simulink model "Q4_Sensor_Unpack"  (R2018b)
settings: Solver=VariableStepAuto  StartTime=0.0  StopTime=10.0  RelTol=1e-3
(part 1 of 2)
settings Model: Creator=82358  LastModifiedBy=82358

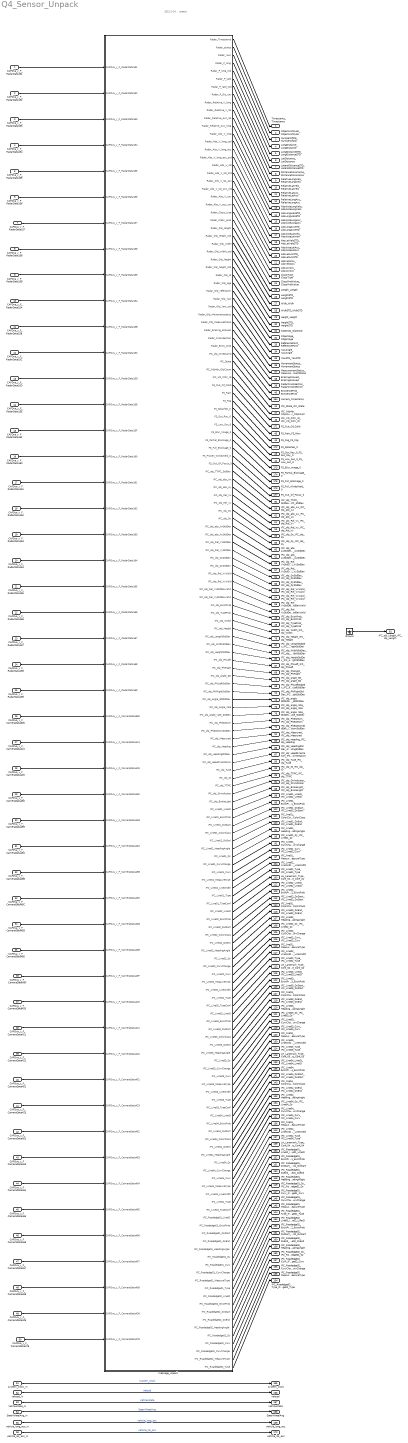
== system Q4_Sensor_Unpack ==
  note: 2021-2-24：unpack
  CAFDva_y_F_RadarData151 : Inport
  CAFDva_y_F_RadarData152 : Inport  Port=2
  CAFDva_y_F_RadarData153 : Inport  Port=3
  CAFDva_y_F_RadarData154 : Inport  Port=4
  CAFDva_y_F_RadarData155 : Inport  Port=5
  CAFDva_y_F_RadarData156 : Inport  Port=6
  CAFDva_y_F_RadarData157 : Inport  Port=7
  CAFDva_y_F_RadarData158 : Inport  Port=8
  CAFDva_y_F_RadarData159 : Inport  Port=9
  CAFDva_y_F_RadarData15A : Inport  Port=10
  CAFDva_y_F_RadarData15B : Inport  Port=11
  CAFDva_y_F_RadarData15C : Inport  Port=12
  CAFDva_y_F_RadarData15D : Inport  Port=13
  CAFDva_y_F_RadarData15E : Inport  Port=14
  CAFDva_y_F_RadarData15F : Inport  Port=15
  CAFDva_y_F_RadarData160 : Inport  Port=16
  CAFDva_y_F_RadarData161 : Inport  Port=17
  CAFDva_y_F_RadarData162 : Inport  Port=18
  CAFDva_y_F_RadarData163 : Inport  Port=19
  CAFDva_y_F_RadarData164 : Inport  Port=20
  CAFDva_y_F_RadarData165 : Inport  Port=21
  CAFDva_y_F_RadarData166 : Inport  Port=22
  CAFDva_y_F_RadarData167 : Inport  Port=23
  CAFDva_y_F_RadarData168 : Inport  Port=24
  CAFDva_y_F_RadarData169 : Inport  Port=25
  CAFDva_y_F_CameraData600 : Inport  Port=26
  CAFDva_y_F_CameraData424 : Inport  Port=27
  CAFDva_y_F_CameraData425 : Inport  Port=28
  CAFDva_y_F_CameraData450 : Inport  Port=29
  CAFDva_y_F_CameraData459 : Inport  Port=30
  CAFDva_y_F_CameraData45A : Inport  Port=31
  CAFDva_y_F_CameraData45B : Inport  Port=32
  CAFDva_y_F_CameraData45C : Inport  Port=33
  CAFDva_y_F_CameraData45D : Inport  Port=34
  CAFDva_y_F_CameraData45E : Inport  Port=35
  CAFDva_y_F_CameraData45F : Inport  Port=36
  CAFDva_y_F_CameraData420 : Inport  Port=37
  CAFDva_y_F_CameraData421 : Inport  Port=38
  CAFDva_y_F_CameraData422 : Inport  Port=39
  CAFDva_y_F_CameraData451 : Inport  Port=40
  CAFDva_y_F_CameraData423 : Inport  Port=41
  CAFDva_y_F_CameraData452 : Inport  Port=42
  CAFDva_y_F_CameraData453 : Inport  Port=43
  CAFDva_y_F_CameraData454 : Inport  Port=44
  CAFDva_y_F_CameraData455 : Inport  Port=45
  CAFDva_y_F_CameraData456 : Inport  Port=46
  CAFDva_y_F_CameraData457 : Inport  Port=47
  CAFDva_y_F_CameraData458 : Inport  Port=48
  CAFDva_y_F_CameraData426 : Inport  Port=49
  CAFDva_y_F_CameraData47E : Inport  Port=50
  system_clock_in : Inport  Port=51  OutDataTypeStr=uint16  PortDimensions=1
  vehspd_in : Inport  Port=52  OutDataTypeStr=T_M_Nm_Float32  PortDimensions=1
  VehYawRate_in : Inport  Port=53  OutDataTypeStr=T_M_Nm_Float32  PortDimensions=1
  SteerWheelAng_in : Inport  Port=54  OutDataTypeStr=T_M_Nm_Float32  PortDimensions=1
  vehicle_long_acc_in : Inport  Port=55  OutDataTypeStr=T_M_Nm_Float32  PortDimensions=1
  vehicle_lat_acc_in : Inport  Port=56  OutDataTypeStr=T_M_Nm_Float32  PortDimensions=1
  Ground : Ground
  message_unpack : MATLAB Function  TreatAsAtomicUnit=on
  Timestamp_Timestamp : Outport
  ObjectListQuali_ObjectListQuali : Outport  Port=2
  NumberOfObj_NumberOfObj : Outport  Port=3
  LongDistance_LongDistance : Outport  Port=4
  LongDistanceSTD_LongDistanceSTD : Outport  Port=5
  LatDistance_LatDistance : Outport  Port=6
  LateralDistanceSTD_LateralDistanceSTD : Outport  Port=7
  DistanceCovariance_DistanceCovariance : Outport  Port=8
  RelativeLongVelo_RelativeLongVelo : Outport  Port=9
  RelativeLatVelo_RelativeLatVelo : Outport  Port=10
  RelativeLatAcc_RelativeLatAcc : Outport  Port=11
  RelativeLongAcc_RelativeLongAcc : Outport  Port=12
  AbsoluteLongVelo_AbsoluteLongVelo : Outport  Port=13
  AbsLongVeloSTD_AbsLongVeloSTD : Outport  Port=14
  AbsoluteLongAcc_AbsoluteLongAcc : Outport  Port=15
  AbsLongAccSTD_AbsLongAccSTD : Outport  Port=16
  AbsoluteLatVelo_AbsoluteLatVelo : Outport  Port=17
  AbsLatVeloSTD_AbsLatVeloSTD : Outport  Port=18
  AbsoluteLatAcc_AbsoluteLatAcc : Outport  Port=19
  AbsLatAccSTD_AbsLatAccSTD : Outport  Port=20
  AbsVeloCov_AbsVeloCov : Outport  Port=21
  AbsAccCov_AbsAccCov : Outport  Port=22
  ClassType_ClassType : Outport  Port=23
  ClassProbValue_ClassProbValue : Outport  Port=24
  Length_Length : Outport  Port=25
  LengthSTD_LengthSTD : Outport  Port=26
  Widh_Widh : Outport  Port=27
  WidhSTD_WidhSTD : Outport  Port=28
  Height_Height : Outport  Port=29
  HeightSTD_HeightSTD : Outport  Port=30
  ObjectID_ObjectID : Outport  Port=31
  ObjectAge_ObjectAge : Outport  Port=32
  ReferencePoint_ReferencePoint : Outport  Port=33
  YawAngle_YawAngle : Outport  Port=34
  YawSTD_YawSTD : Outport  Port=35
  MovementStatus_MovementStatus : Outport  Port=36
  MeasurementStatus_MeasurementStatus : Outport  Port=37
  BrakingAllowed_BrakingAllowed : Outport  Port=38
  RadarCrossSection_RadarCrossSection : Outport  Port=39
  ExistenceProb_ExistenceProb : Outport  Port=40
  IFC_State_IFC_State : Outport  Port=41
  FS_Low_Sun_0_FS_Low_Sun_0 : Outport  Port=42
  FS_Sun_Ray_0_FS_Sun_Ray_0 : Outport  Port=43
  FS_Fog_FS_Fog : Outport  Port=44
  FS_Rain_FS_Rain : Outport  Port=45
  IFC_VD_CIPV_ID_IFC_VD_CIPV_ID : Outport  Port=46
  IFC_ObjHdr_ObjCount_IFC_ObjHdr_ObjCount : Outport  Port=47
  IFC_obj_ExistProb_IFC_obj_ExistProb : Outport  Port=48
  IFC_obj_TypeProb_IFC_obj_TypeProb : Outport  Port=49
  IFC_obj_Type_IFC_obj_Type : Outport  Port=50
  IFC_obj_Rel_Vx_IFC_obj_Rel_Vx : Outport  Port=51
  IFC_obj_Rel_VxValid_IFC_obj_Rel_VxValid : Outport  Port=52
  IFC_obj_Rel_Vy_IFC_obj_Rel_Vy : Outport  Port=53
  IFC_obj_Rel_VyValid_IFC_obj_Rel_VyValid : Outport  Port=54
  IFC_obj_Rel_VxStdDev_IFC_obj_Rel_VxStdDev : Outport  Port=55
  IFC_obj_Rel_VxStdDevValid_IFC_obj_Rel_VxStdDevValid : Outport  Port=56
  IFC_obj_Rel_VyStdDev_IFC_obj_Rel_VyStdDev : Outport  Port=57
  IFC_obj_Rel_VyStdDevValid_IFC_obj_Rel_VyStdDevValid : Outport  Port=58
  IFC_obj_abs_Ax_IFC_obj_abs_Ax : Outport  Port=59
  IFC_obj_abs_AxStdDev_IFC_obj_abs_AxStdDev : Outport  Port=60
  IFC_obj_abs_Ay_IFC_obj_abs_Ay : Outport  Port=61
  IFC_obj_abs_AyStdDev_IFC_obj_abs_AyStdDev : Outport  Port=62
  IFC_obj_Dx_IFC_obj_Dx : Outport  Port=63
  IFC_obj_DxStdDev_IFC_obj_DxStdDev : Outport  Port=64
  IFC_obj_Dy_IFC_obj_Dy : Outport  Port=65
  IFC_obj_DyStdDev_IFC_obj_DyStdDev : Outport  Port=66
  IFC_obj_PhiLeft_IFC_obj_PhiLeft : Outport  Port=67
  IFC_obj_PhiLeftStdDev_IFC_obj_PhiLeftStdDev : Outport  Port=68
  IFC_obj_PhiRight_IFC_obj_PhiRight : Outport  Port=69
  IFC_obj_PhiRightStdDev_IFC_obj_PhiRightStdDev : Outport  Port=70
  IFC_obj_PhiBottom_IFC_obj_PhiBottom : Outport  Port=71
  IFC_obj_PhiBottomStdDev_IFC_obj_PhiBottomStdDev : Outport  Port=72
  IFC_obj_angle_3D_IFC_obj_angle_3D : Outport  Port=73
  IFC_obj_angle_3DStdDev_IFC_obj_angle_3DStdDev : Outport  Port=74
  IFC_obj_angle_rate_IFC_obj_angle_rate : Outport  Port=75
  IFC_obj_angle_rate_StdDev_IFC_obj_angle_rate_StdDev : Outport  Port=76
  IFC_obj_Width_IFC_obj_Width : Outport  Port=77
  IFC_obj_WidthStdDev_IFC_obj_WidthStdDev : Outport  Port=78
  IFC_obj_Height_IFC_obj_Height : Outport  Port=79
  IFC_obj_HeightStdDev_IFC_obj_HeightStdDev : Outport  Port=80
  IFC_obj_Length_IFC_obj_Length : Outport  Port=81  OutDataTypeStr=single  PortDimensions=20  SampleTime=0.06
  IFC_obj_LengthStdDev_IFC_obj_LengthStdDev : Outport  Port=82
  IFC_obj_ID_IFC_obj_ID : Outport  Port=83
  IFC_obj_DirIndicator_IFC_obj_DirIndicator : Outport  Port=84
  IFC_obj_Heading_IFC_obj_Heading : Outport  Port=85
  IFC_obj_HeadingStdDev_IFC_obj_HeadingStdDev : Outport  Port=86
  IFC_obj_HeadOrientation_IFC_obj_HeadOrientation : Outport  Port=87
  IFC_obj_BrakeLight_IFC_obj_BrakeLight : Outport  Port=88
  IFC_obj_TTIPC_IFC_obj_TTIPC : Outport  Port=89
  IFC_obj_TTIPC_StdDev_IFC_obj_TTIPC_StdDev : Outport  Port=90
  IFC_obj_Measured_IFC_obj_Measured : Outport  Port=91
  IFC_Line01_CurvChange_IFC_Line01_CurvChange : Outport  Port=92
  IFC_Line01_Curv_IFC_Line01_Curv : Outport  Port=93
  IFC_Line01_HeadingAngle_IFC_Line01_HeadingAngle : Outport  Port=94
  IFC_Line01_Dy_IFC_Line01_Dy : Outport  Port=95
  IFC_Line01_ExistProb_IFC_Line01_ExistProb : Outport  Port=96
  IFC_line01_MeasureType_IFC_line01_MeasureType : Outport  Port=97
  IFC_Line01_Type_IFC_Line01_Type : Outport  Port=98
  IFC_Line01_LineID_IFC_Line01_LineID : Outport  Port=99
  LH_Lanemark_Type_Conf_01_LH_Lanemark_Type_Conf_01 : Outport  Port=100
  IFC_line01_ColorClass_IFC_line01_ColorClass : Outport  Port=101
  IFC_Line01_DxStart_IFC_Line01_DxStart : Outport  Port=102
  IFC_Line01_DxEnd_IFC_Line01_DxEnd : Outport  Port=103
  IFC_Line01_LineWidth_IFC_Line01_LineWidth : Outport  Port=104
  IFC_Line02_CurvChange_IFC_Line02_CurvChange : Outport  Port=105
  IFC_Line02_Curv_IFC_Line02_Curv : Outport  Port=106
  IFC_Line02_HeadingAngle_IFC_Line02_HeadingAngle : Outport  Port=107
  IFC_Line02_Dy_IFC_Line02_Dy : Outport  Port=108
  IFC_Line02_ExistProb_IFC_Line02_ExistProb : Outport  Port=109
  IFC_line02_MeasureType_IFC_line02_MeasureType : Outport  Port=110
  IFC_Line02_Type_IFC_Line02_Type : Outport  Port=111
  IFC_Line02_LineID_IFC_Line02_LineID : Outport  Port=112
  LH_Lanemark_Type_Conf_02_LH_Lanemark_Type_Conf_02 : Outport  Port=113
  IFC_line02_ColorClass_IFC_line02_ColorClass : Outport  Port=114
  IFC_Line02_DxStart_IFC_Line02_DxStart : Outport  Port=115
  IFC_Line02_DxEnd_IFC_Line02_DxEnd : Outport  Port=116
  IFC_Line02_LineWidth_IFC_Line02_LineWidth : Outport  Port=117
  IFC_Line03_CurvChange_IFC_Line03_CurvChange : Outport  Port=118
  IFC_Line03_Curv_IFC_Line03_Curv : Outport  Port=119
  IFC_Line03_HeadingAngle_IFC_Line03_HeadingAngle : Outport  Port=120
  IFC_Line03_Dy_IFC_Line03_Dy : Outport  Port=121
  IFC_Line03_ExistProb_IFC_Line03_ExistProb : Outport  Port=122
  IFC_line03_MeasureType_IFC_line03_MeasureType : Outport  Port=123
  IFC_Line03_Type_IFC_Line03_Type : Outport  Port=124
  IFC_Line03_LineID_IFC_Line03_LineID : Outport  Port=125
  LH_Lanemark_Type_Conf_03_LH_Lanemark_Type_Conf_03 : Outport  Port=126
  IFC_line03_ColorClass_IFC_line03_ColorClass : Outport  Port=127
  IFC_Line03_DxStart_IFC_Line03_DxStart : Outport  Port=128
  IFC_Line03_DxEnd_IFC_Line03_DxEnd : Outport  Port=129
  IFC_Line03_LineWidth_IFC_Line03_LineWidth : Outport  Port=130
  IFC_Line04_CurvChange_IFC_Line04_CurvChange : Outport  Port=131
  IFC_Line04_Curv_IFC_Line04_Curv : Outport  Port=132
  IFC_Line04_HeadingAngle_IFC_Line04_HeadingAngle : Outport  Port=133
  IFC_Line04_Dy_IFC_Line04_Dy : Outport  Port=134
  IFC_Line04_ExistProb_IFC_Line04_ExistProb : Outport  Port=135
  IFC_line04_MeasureType_IFC_line04_MeasureType : Outport  Port=136
  IFC_Line04_Type_IFC_Line04_Type : Outport  Port=137
  IFC_Line04_LineID_IFC_Line04_LineID : Outport  Port=138
  LH_Lanemark_Type_Conf_04_LH_Lanemark_Type_Conf_04 : Outport  Port=139
  IFC_line04_ColorClass_IFC_line04_ColorClass : Outport  Port=140
  IFC_Line04_DxStart_IFC_Line04_DxStart : Outport  Port=141
  IFC_Line04_DxEnd_IFC_Line04_DxEnd : Outport  Port=142
  IFC_Line04_LineWidth_IFC_Line04_LineWidth : Outport  Port=143
  IFC_Roadedge01_Type_IFC_Roadedge01_Type : Outport  Port=144
  IFC_Roadedge01_MeasureType_IFC_Roadedge01_MeasureType : Outport  Port=145
  IFC_Roadedge01_CurvChange_IFC_Roadedge01_CurvChange : Outport  Port=146
  IFC_Roadedge01_Curv_IFC_Roadedge01_Curv : Outport  Port=147
  IFC_Roadedge01_HeadingAngle_IFC_Roadedge01_HeadingAngle : Outport  Port=148
  IFC_Roadedge01_Dy_IFC_Roadedge01_Dy : Outport  Port=149
  IFC_Roadedge01_DxEnd_IFC_Roadedge01_DxEnd : Outport  Port=150
  IFC_Roadedge01_DxStart_IFC_Roadedge01_DxStart : Outport  Port=151
  IFC_Roadedge01_ExistProb_IFC_Roadedge01_ExistProb : Outport  Port=152
  IFC_Roadedge01_LineID_IFC_Roadedge01_LineID : Outport  Port=153
  IFC_Roadedge02_Type_IFC_Roadedge02_Type : Outport  Port=154
  IFC_Roadedge02_MeasureType_IFC_Roadedge02_MeasureType : Outport  Port=155
  IFC_Roadedge02_CurvChange_IFC_Roadedge02_CurvChange : Outport  Port=156
  IFC_Roadedge02_Curv_IFC_Roadedge02_Curv : Outport  Port=157
  IFC_Roadedge02_HeadingAngle_IFC_Roadedge02_HeadingAngle : Outport  Port=158
  IFC_Roadedge02_Dy_IFC_Roadedge02_Dy : Outport  Port=159
  IFC_Roadedge02_DxEnd_IFC_Roadedge02_DxEnd : Outport  Port=160
  IFC_Roadedge02_DxStart_IFC_Roadedge02_DxStart : Outport  Port=161
  IFC_Roadedge02_ExistProb_IFC_Roadedge02_ExistProb : Outport  Port=162
  IFC_Roadedge02_LineID_IFC_Roadedge02_LineID : Outport  Port=163
  camera_timestamp : Outport  Port=164
  system_clock : Outport  Port=165
  vehspd : Outport  Port=166
  VehYawRate : Outport  Port=167
  SteerWheelAng : Outport  Port=168
  vehicle_long_acc : Outport  Port=169
  vehicle_lat_acc : Outport  Port=170
  FS_Out_Of_Calib : Outport  Port=171
  FS_Splashes_0 : Outport  Port=172
  FS_Blur_Image_0 : Outport  Port=173
  FS_Partial_Blockage_0 : Outport  Port=174
  FS_Full_Blockage_0 : Outport  Port=175
  FS_Full_Windshield_0 : Outport  Port=176
  FS_Out_Of_Focus_0 : Outport  Port=177
  wires:
  CAFDva_y_F_RadarData161/1 -> message_unpack/17(CAFDva_y_F_RadarData161)
  message_unpack/162(IFC_Roadedge02_ExistProb) -> IFC_Roadedge02_ExistProb_IFC_Roadedge02_ExistProb/1
  message_unpack/1(Radar_Timestamp) -> Timestamp_Timestamp/1
  message_unpack/168(IFC_Roadedge02_CurvChange) -> IFC_Roadedge02_CurvChange_IFC_Roadedge02_CurvChange/1
  CAFDva_y_F_CameraData45A/1 -> message_unpack/31(CAFDva_y_F_CameraData45A)
  message_unpack/30(Radar_Obj_height_std) -> HeightSTD_HeightSTD/1
  message_unpack/79(IFC_obj_HeightStdDev) -> IFC_obj_HeightStdDev_IFC_obj_HeightStdDev/1
  CAFDva_y_F_RadarData15B/1 -> message_unpack/11(CAFDva_y_F_RadarData15B)
  message_unpack/78(IFC_obj_WidthStdDev) -> IFC_obj_WidthStdDev_IFC_obj_WidthStdDev/1
  message_unpack/61(IFC_obj_Dx) -> IFC_obj_Dx_IFC_obj_Dx/1
  CAFDva_y_F_RadarData169/1 -> message_unpack/25(CAFDva_y_F_RadarData169)
  message_unpack/70(IFC_obj_Rel_VyValid) -> IFC_obj_Rel_VyValid_IFC_obj_Rel_VyValid/1
  CAFDva_y_F_RadarData159/1 -> message_unpack/9(CAFDva_y_F_RadarData159)
  message_unpack/68(IFC_obj_DyStdDev) -> IFC_obj_DyStdDev_IFC_obj_DyStdDev/1
  message_unpack/62(IFC_obj_Dy) -> IFC_obj_Dy_IFC_obj_Dy/1
  message_unpack/166(IFC_Roadedge02_Dy) -> IFC_Roadedge02_Dy_IFC_Roadedge02_Dy/1
  message_unpack/54(FS_Frozen_Windshield_0) -> FS_Full_Windshield_0/1
  message_unpack/88(IFC_obj_PhiBottom) -> IFC_obj_PhiBottom_IFC_obj_PhiBottom/1
  message_unpack/50(FS_Low_Sun_0) -> FS_Low_Sun_0_FS_Low_Sun_0/1
  message_unpack/52(FS_Partial_Blockage_0) -> FS_Partial_Blockage_0/1
  message_unpack/45(FS_Out_Of_Calib) -> FS_Out_Of_Calib/1
  message_unpack/42(IFC_State) -> IFC_State_IFC_State/1
  message_unpack/49(FS_Sun_Ray_0) -> FS_Sun_Ray_0_FS_Sun_Ray_0/1
  CAFDva_y_F_CameraData600/1 -> message_unpack/26(CAFDva_y_F_CameraData600)
  CAFDva_y_F_RadarData154/1 -> message_unpack/4(CAFDva_y_F_RadarData154)
  message_unpack/34(Radar_Obj_Yaw) -> YawAngle_YawAngle/1
  message_unpack/12(Radar_Relative_Acc_long) -> RelativeLongAcc_RelativeLongAcc/1
  vehspd_in/1 -> vehspd/1  "vehspd"
  message_unpack/8(Radar_P_Dis_cov) -> DistanceCovariance_DistanceCovariance/1
  message_unpack/24(Radar_Class_prob) -> ClassProbValue_ClassProbValue/1
  system_clock_in/1 -> system_clock/1  "system_clock"
  SteerWheelAng_in/1 -> SteerWheelAng/1  "SteerWheelAng"
  CAFDva_y_F_CameraData421/1 -> message_unpack/38(CAFDva_y_F_CameraData421)
  CAFDva_y_F_RadarData168/1 -> message_unpack/24(CAFDva_y_F_RadarData168)
  CAFDva_y_F_CameraData424/1 -> message_unpack/27(CAFDva_y_F_CameraData424)
  CAFDva_y_F_RadarData151/1 -> message_unpack/1(CAFDva_y_F_RadarData151)
  message_unpack/56(IFC_obj_TTIPC_StdDev) -> IFC_obj_TTIPC_StdDev_IFC_obj_TTIPC_StdDev/1
  message_unpack/114(IFC_Line02_DxStart) -> IFC_Line02_DxStart_IFC_Line02_DxStart/1
  CAFDva_y_F_CameraData45B/1 -> message_unpack/32(CAFDva_y_F_CameraData45B)
  message_unpack/156(IFC_Roadedge01_Dy) -> IFC_Roadedge01_Dy_IFC_Roadedge01_Dy/1
  message_unpack/102(IFC_Line01_ColorClass) -> IFC_line01_ColorClass_IFC_line01_ColorClass/1
  message_unpack/25(Radar_Obj_length) -> Length_Length/1
  message_unpack/108(IFC_Line01_MeasureType) -> IFC_line01_MeasureType_IFC_line01_MeasureType/1
  message_unpack/152(IFC_Roadedge01_ExistProb) -> IFC_Roadedge01_ExistProb_IFC_Roadedge01_ExistProb/1
  message_unpack/91(IFC_obj_Heading) -> IFC_obj_Heading_IFC_obj_Heading/1
  message_unpack/60(IFC_obj_Rel_Vy) -> IFC_obj_Rel_Vy_IFC_obj_Rel_Vy/1
  message_unpack/126(IFC_Line03_ExistProb) -> IFC_Line03_ExistProb_IFC_Line03_ExistProb/1
  CAFDva_y_F_CameraData451/1 -> message_unpack/40(CAFDva_y_F_CameraData451)
  message_unpack/146(IFC_Line04_Curv) -> IFC_Line04_Curv_IFC_Line04_Curv/1
  message_unpack/101(IFC_Line01_DxStart) -> IFC_Line01_DxStart_IFC_Line01_DxStart/1
  message_unpack/113(IFC_Line02_ExistProb) -> IFC_Line02_ExistProb_IFC_Line02_ExistProb/1
  message_unpack/89(IFC_obj_PhiBottomStdDev) -> IFC_obj_PhiBottomStdDev_IFC_obj_PhiBottomStdDev/1
  message_unpack/46(FS_Rain) -> FS_Rain_FS_Rain/1
  message_unpack/106(IFC_Line01_CurvChange) -> IFC_Line01_CurvChange_IFC_Line01_CurvChange/1
  message_unpack/107(IFC_Line01_Curv) -> IFC_Line01_Curv_IFC_Line01_Curv/1
  message_unpack/66(IFC_obj_Rel_VyStdDev) -> IFC_obj_Rel_VyStdDev_IFC_obj_Rel_VyStdDev/1
  message_unpack/129(IFC_Line03_DxEnd) -> IFC_Line03_DxEnd_IFC_Line03_DxEnd/1
  message_unpack/109(IFC_Line01_LineWidth) -> IFC_Line01_LineWidth_IFC_Line01_LineWidth/1
  CAFDva_y_F_CameraData458/1 -> message_unpack/48(CAFDva_y_F_CameraData458)
  message_unpack/111(IFC_Line01_TypeConf) -> LH_Lanemark_Type_Conf_01_LH_Lanemark_Type_Conf_01/1
  message_unpack/137(IFC_Line03_TypeConf) -> LH_Lanemark_Type_Conf_03_LH_Lanemark_Type_Conf_03/1
  message_unpack/17(Radar_Abs_V_lat) -> AbsoluteLatVelo_AbsoluteLatVelo/1
  CAFDva_y_F_RadarData166/1 -> message_unpack/22(CAFDva_y_F_RadarData166)
  message_unpack/112(IFC_Line02_LineID) -> IFC_Line02_LineID_IFC_Line02_LineID/1
  message_unpack/115(IFC_Line02_ColorClass) -> IFC_line02_ColorClass_IFC_line02_ColorClass/1
  message_unpack/110(IFC_Line01_Type) -> IFC_Line01_Type_IFC_Line01_Type/1
  message_unpack/73(IFC_obj_ExistProb) -> IFC_obj_ExistProb_IFC_obj_ExistProb/1
  message_unpack/116(IFC_Line02_DxEnd) -> IFC_Line02_DxEnd_IFC_Line02_DxEnd/1
  CAFDva_y_F_CameraData452/1 -> message_unpack/42(CAFDva_y_F_CameraData452)
  message_unpack/74(IFC_obj_TypeProb) -> IFC_obj_TypeProb_IFC_obj_TypeProb/1
  message_unpack/20(Radar_Abs_V_lat_acc_std) -> AbsLatAccSTD_AbsLatAccSTD/1
  message_unpack/123(IFC_Line02_Type) -> IFC_Line02_Type_IFC_Line02_Type/1
  message_unpack/47(FS_Fog) -> FS_Fog_FS_Fog/1
  CAFDva_y_F_CameraData47E/1 -> message_unpack/50(CAFDva_y_F_CameraData47E)
  message_unpack/117(IFC_Line02_HeadingAngle) -> IFC_Line02_HeadingAngle_IFC_Line02_HeadingAngle/1
  CAFDva_y_F_RadarData162/1 -> message_unpack/18(CAFDva_y_F_RadarData162)
  message_unpack/159(IFC_Roadedge01_MeasureType) -> IFC_Roadedge01_MeasureType_IFC_Roadedge01_MeasureType/1
  message_unpack/43(IFC_ObjHdr_ObjCount) -> IFC_ObjHdr_ObjCount_IFC_ObjHdr_ObjCount/1
  message_unpack/118(IFC_Line02_Dy) -> IFC_Line02_Dy_IFC_Line02_Dy/1
  CAFDva_y_F_RadarData156/1 -> message_unpack/6(CAFDva_y_F_RadarData156)
  message_unpack/134(IFC_Line03_MeasureType) -> IFC_line03_MeasureType_IFC_line03_MeasureType/1
  message_unpack/145(IFC_Line04_CurvChange) -> IFC_Line04_CurvChange_IFC_Line04_CurvChange/1
  message_unpack/125(IFC_Line03_LineID) -> IFC_Line03_LineID_IFC_Line03_LineID/1
  message_unpack/10(Radar_Relative_V_lat) -> RelativeLatVelo_RelativeLatVelo/1
  message_unpack/119(IFC_Line02_CurvChange) -> IFC_Line02_CurvChange_IFC_Line02_CurvChange/1
  CAFDva_y_F_CameraData45F/1 -> message_unpack/36(CAFDva_y_F_CameraData45F)
  message_unpack/71(IFC_obj_Rel_VxStdDevValid) -> IFC_obj_Rel_VxStdDevValid_IFC_obj_Rel_VxStdDevValid/1
  message_unpack/164(IFC_Roadedge02_DxEnd) -> IFC_Roadedge02_DxEnd_IFC_Roadedge02_DxEnd/1
  message_unpack/140(IFC_Line04_DxStart) -> IFC_Line04_DxStart_IFC_Line04_DxStart/1
  message_unpack/41(IFC_obj_timestamp) -> camera_timestamp/1
  message_unpack/121(IFC_Line02_MeasureType) -> IFC_line02_MeasureType_IFC_line02_MeasureType/1
  message_unpack/99(IFC_Line01_LineID) -> IFC_Line01_LineID_IFC_Line01_LineID/1
  message_unpack/122(IFC_Line02_LineWidth) -> IFC_Line02_LineWidth_IFC_Line02_LineWidth/1
  message_unpack/136(IFC_Line03_Type) -> IFC_Line03_Type_IFC_Line03_Type/1
  message_unpack/133(IFC_Line03_Curv) -> IFC_Line03_Curv_IFC_Line03_Curv/1
  message_unpack/128(IFC_Line03_ColorClass) -> IFC_line03_ColorClass_IFC_line03_ColorClass/1
  message_unpack/124(IFC_Line02_TypeConf) -> LH_Lanemark_Type_Conf_02_LH_Lanemark_Type_Conf_02/1
  message_unpack/92(IFC_obj_HeadingStdDev) -> IFC_obj_HeadingStdDev_IFC_obj_HeadingStdDev/1
  CAFDva_y_F_CameraData454/1 -> message_unpack/44(CAFDva_y_F_CameraData454)
  CAFDva_y_F_CameraData420/1 -> message_unpack/37(CAFDva_y_F_CameraData420)
  message_unpack/132(IFC_Line03_CurvChange) -> IFC_Line03_CurvChange_IFC_Line03_CurvChange/1
  message_unpack/29(Radar_Obj_height) -> Height_Height/1
  message_unpack/55(FS_Out_Of_Focus_0) -> FS_Out_Of_Focus_0/1
  message_unpack/67(IFC_obj_DxStdDev) -> IFC_obj_DxStdDev_IFC_obj_DxStdDev/1
  message_unpack/135(IFC_Line03_LineWidth) -> IFC_Line03_LineWidth_IFC_Line03_LineWidth/1
  message_unpack/150(IFC_Line04_TypeConf) -> LH_Lanemark_Type_Conf_04_LH_Lanemark_Type_Conf_04/1
  message_unpack/151(IFC_Roadedge01_LineID) -> IFC_Roadedge01_LineID_IFC_Roadedge01_LineID/1
  message_unpack/75(IFC_obj_Width) -> IFC_obj_Width_IFC_obj_Width/1
  message_unpack/165(IFC_Roadedge02_HeadingAngle) -> IFC_Roadedge02_HeadingAngle_IFC_Roadedge02_HeadingAngle/1
  message_unpack/170(IFC_Roadedge02_Type) -> IFC_Roadedge02_Type_IFC_Roadedge02_Type/1
  CAFDva_y_F_RadarData15C/1 -> message_unpack/12(CAFDva_y_F_RadarData15C)
  CAFDva_y_F_CameraData426/1 -> message_unpack/49(CAFDva_y_F_CameraData426)
  message_unpack/48(FS_Splashes_0) -> FS_Splashes_0/1
  message_unpack/141(IFC_Line04_ColorClass) -> IFC_line04_ColorClass_IFC_line04_ColorClass/1
  CAFDva_y_F_RadarData158/1 -> message_unpack/8(CAFDva_y_F_RadarData158)
  CAFDva_y_F_RadarData164/1 -> message_unpack/20(CAFDva_y_F_RadarData164)
  message_unpack/37(Radar_Obj_Measurestatus) -> MeasurementStatus_MeasurementStatus/1
  message_unpack/160(IFC_Roadedge01_Type) -> IFC_Roadedge01_Type_IFC_Roadedge01_Type/1
  CAFDva_y_F_RadarData15A/1 -> message_unpack/10(CAFDva_y_F_RadarData15A)
  message_unpack/142(IFC_Line04_DxEnd) -> IFC_Line04_DxEnd_IFC_Line04_DxEnd/1
  message_unpack/82(IFC_obj_angle_3D) -> IFC_obj_angle_3D_IFC_obj_angle_3D/1
  message_unpack/144(IFC_Line04_Dy) -> IFC_Line04_Dy_IFC_Line04_Dy/1
  CAFDva_y_F_RadarData157/1 -> message_unpack/7(CAFDva_y_F_RadarData157)
  message_unpack/28(Radar_Obj_width_std) -> WidhSTD_WidhSTD/1
  message_unpack/69(IFC_obj_Rel_VxValid) -> IFC_obj_Rel_VxValid_IFC_obj_Rel_VxValid/1
  CAFDva_y_F_CameraData455/1 -> message_unpack/45(CAFDva_y_F_CameraData455)
  message_unpack/147(IFC_Line04_MeasureType) -> IFC_line04_MeasureType_IFC_line04_MeasureType/1
  message_unpack/149(IFC_Line04_Type) -> IFC_Line04_Type_IFC_Line04_Type/1
  message_unpack/104(IFC_Line01_HeadingAngle) -> IFC_Line01_HeadingAngle_IFC_Line01_HeadingAngle/1
  message_unpack/158(IFC_Roadedge01_CurvChange) -> IFC_Roadedge01_CurvChange_IFC_Roadedge01_CurvChange/1
  message_unpack/23(Radar_Class_type) -> ClassType_ClassType/1
  message_unpack/157(IFC_Roadedge01_Curv) -> IFC_Roadedge01_Curv_IFC_Roadedge01_Curv/1
  message_unpack/87(IFC_obj_angle_rate_StdDev) -> IFC_obj_angle_rate_StdDev_IFC_obj_angle_rate_StdDev/1
  message_unpack/44(IFC_VD_CIPV_ID) -> IFC_VD_CIPV_ID_IFC_VD_CIPV_ID/1
  message_unpack/169(IFC_Roadedge02_MeasureType) -> IFC_Roadedge02_MeasureType_IFC_Roadedge02_MeasureType/1
  message_unpack/76(IFC_obj_Height) -> IFC_obj_Height_IFC_obj_Height/1
  CAFDva_y_F_CameraData45D/1 -> message_unpack/34(CAFDva_y_F_CameraData45D)
  message_unpack/161(IFC_Roadedge02_LineID) -> IFC_Roadedge02_LineID_IFC_Roadedge02_LineID/1
  message_unpack/15(Radar_Abs_V_long_acc) -> AbsoluteLongAcc_AbsoluteLongAcc/1
  message_unpack/22(Radar_Abs_V_acc_cov) -> AbsAccCov_AbsAccCov/1
  message_unpack/9(Radar_Relative_V_long) -> RelativeLongVelo_RelativeLongVelo/1
  message_unpack/18(Radar_Abs_V_lat_std) -> AbsLatVeloSTD_AbsLatVeloSTD/1
  message_unpack/40(Radar_Exist_prob) -> ExistenceProb_ExistenceProb/1
  message_unpack/19(Radar_Abs_V_lat_acc) -> AbsoluteLatAcc_AbsoluteLatAcc/1
  CAFDva_y_F_RadarData160/1 -> message_unpack/16(CAFDva_y_F_RadarData160)
  message_unpack/11(Radar_Relative_Acc_lat) -> RelativeLatAcc_RelativeLatAcc/1
  message_unpack/16(Radar_Abs_V_long_acc_std) -> AbsLongAccSTD_AbsLongAccSTD/1
  message_unpack/31(Radar_Obj_id) -> ObjectID_ObjectID/1
  message_unpack/155(IFC_Roadedge01_HeadingAngle) -> IFC_Roadedge01_HeadingAngle_IFC_Roadedge01_HeadingAngle/1
  CAFDva_y_F_CameraData453/1 -> message_unpack/43(CAFDva_y_F_CameraData453)
  message_unpack/21(Radar_Abs_V_cov) -> AbsVeloCov_AbsVeloCov/1
  message_unpack/77(IFC_obj_LengthStdDev) -> IFC_obj_LengthStdDev_IFC_obj_LengthStdDev/1
  CAFDva_y_F_CameraData423/1 -> message_unpack/41(CAFDva_y_F_CameraData423)
  CAFDva_y_F_RadarData152/1 -> message_unpack/2(CAFDva_y_F_RadarData152)
  vehicle_lat_acc_in/1 -> vehicle_lat_acc/1  "vehicle_lat_acc"
  message_unpack/33(Radar_Obj_referpoint) -> ReferencePoint_ReferencePoint/1
  message_unpack/53(FS_Full_Blockage_0) -> FS_Full_Blockage_0/1
  CAFDva_y_F_RadarData165/1 -> message_unpack/21(CAFDva_y_F_RadarData165)
  message_unpack/83(IFC_obj_PhiLeftStdDev) -> IFC_obj_PhiLeftStdDev_IFC_obj_PhiLeftStdDev/1
  CAFDva_y_F_RadarData167/1 -> message_unpack/23(CAFDva_y_F_RadarData167)
  message_unpack/7(Radar_P_latd_std) -> LateralDistanceSTD_LateralDistanceSTD/1
  message_unpack/72(IFC_obj_Rel_VyStdDevValid) -> IFC_obj_Rel_VyStdDevValid_IFC_obj_Rel_VyStdDevValid/1
  message_unpack/13(Radar_Abs_V_long) -> AbsoluteLongVelo_AbsoluteLongVelo/1
  CAFDva_y_F_CameraData45E/1 -> message_unpack/35(CAFDva_y_F_CameraData45E)
  message_unpack/38(Radar_Braking_allowed) -> BrakingAllowed_BrakingAllowed/1
  message_unpack/153(IFC_Roadedge01_DxStart) -> IFC_Roadedge01_DxStart_IFC_Roadedge01_DxStart/1
  message_unpack/167(IFC_Roadedge02_Curv) -> IFC_Roadedge02_Curv_IFC_Roadedge02_Curv/1
  message_unpack/154(IFC_Roadedge01_DxEnd) -> IFC_Roadedge01_DxEnd_IFC_Roadedge01_DxEnd/1
  Ground/1 -> IFC_obj_Length_IFC_obj_Length/1
  message_unpack/80(IFC_obj_PhiLeft) -> IFC_obj_PhiLeft_IFC_obj_PhiLeft/1
  CAFDva_y_F_CameraData422/1 -> message_unpack/39(CAFDva_y_F_CameraData422)
  message_unpack/2(Radar_status) -> ObjectListQuali_ObjectListQuali/1
  message_unpack/32(Radar_Obj_age) -> ObjectAge_ObjectAge/1
  VehYawRate_in/1 -> VehYawRate/1  "VehYawRate"
  CAFDva_y_F_CameraData456/1 -> message_unpack/46(CAFDva_y_F_CameraData456)
  message_unpack/35(Radar_Obj_Yaw_std) -> YawSTD_YawSTD/1
  message_unpack/59(IFC_obj_Rel_Vx) -> IFC_obj_Rel_Vx_IFC_obj_Rel_Vx/1
  message_unpack/84(IFC_obj_PhiRightStdDev) -> IFC_obj_PhiRightStdDev_IFC_obj_PhiRightStdDev/1
  message_unpack/143(IFC_Line04_HeadingAngle) -> IFC_Line04_HeadingAngle_IFC_Line04_HeadingAngle/1
  CAFDva_y_F_RadarData15D/1 -> message_unpack/13(CAFDva_y_F_RadarData15D)
  message_unpack/93(IFC_obj_HeadOrientation) -> IFC_obj_HeadOrientation_IFC_obj_HeadOrientation/1
  message_unpack/26(Radar_Obj_length_std) -> LengthSTD_LengthSTD/1
  CAFDva_y_F_CameraData457/1 -> message_unpack/47(CAFDva_y_F_CameraData457)
  message_unpack/27(Radar_Obj_width) -> Widh_Widh/1
  CAFDva_y_F_RadarData15F/1 -> message_unpack/15(CAFDva_y_F_RadarData15F)
  message_unpack/57(IFC_obj_abs_Ax) -> IFC_obj_abs_Ax_IFC_obj_abs_Ax/1
  message_unpack/98(IFC_obj_BrakeLight) -> IFC_obj_BrakeLight_IFC_obj_BrakeLight/1
  message_unpack/63(IFC_obj_abs_AxStdDev) -> IFC_obj_abs_AxStdDev_IFC_obj_abs_AxStdDev/1
  CAFDva_y_F_RadarData153/1 -> message_unpack/3(CAFDva_y_F_RadarData153)
  CAFDva_y_F_CameraData459/1 -> message_unpack/30(CAFDva_y_F_CameraData459)
  CAFDva_y_F_RadarData163/1 -> message_unpack/19(CAFDva_y_F_RadarData163)
  message_unpack/90(IFC_obj_Measured) -> IFC_obj_Measured_IFC_obj_Measured/1
  message_unpack/148(IFC_Line04_LineWidth) -> IFC_Line04_LineWidth_IFC_Line04_LineWidth/1
  CAFDva_y_F_RadarData15E/1 -> message_unpack/14(CAFDva_y_F_RadarData15E)
  message_unpack/39(Radar_CrossSection) -> RadarCrossSection_RadarCrossSection/1
  message_unpack/139(IFC_Line04_ExistProb) -> IFC_Line04_ExistProb_IFC_Line04_ExistProb/1
  message_unpack/65(IFC_obj_Rel_VxStdDev) -> IFC_obj_Rel_VxStdDev_IFC_obj_Rel_VxStdDev/1
  message_unpack/138(IFC_Line04_LineID) -> IFC_Line04_LineID_IFC_Line04_LineID/1
  CAFDva_y_F_CameraData45C/1 -> message_unpack/33(CAFDva_y_F_CameraData45C)
  message_unpack/64(IFC_obj_abs_AyStdDev) -> IFC_obj_abs_AyStdDev_IFC_obj_abs_AyStdDev/1
  message_unpack/81(IFC_obj_PhiRight) -> IFC_obj_PhiRight_IFC_obj_PhiRight/1
  message_unpack/14(Radar_Abs_V_long_std) -> AbsLongVeloSTD_AbsLongVeloSTD/1
  message_unpack/127(IFC_Line03_DxStart) -> IFC_Line03_DxStart_IFC_Line03_DxStart/1
  message_unpack/86(IFC_obj_angle_rate) -> IFC_obj_angle_rate_IFC_obj_angle_rate/1
  message_unpack/100(IFC_Line01_ExistProb) -> IFC_Line01_ExistProb_IFC_Line01_ExistProb/1
  message_unpack/94(IFC_obj_Type) -> IFC_obj_Type_IFC_obj_Type/1
  message_unpack/85(IFC_obj_angle_3DStdDev) -> IFC_obj_angle_3DStdDev_IFC_obj_angle_3DStdDev/1
  message_unpack/95(IFC_obj_ID) -> IFC_obj_ID_IFC_obj_ID/1
  CAFDva_y_F_RadarData155/1 -> message_unpack/5(CAFDva_y_F_RadarData155)
  message_unpack/4(Radar_P_long) -> LongDistance_LongDistance/1
  message_unpack/36(Radar_Obj_Movementstatus) -> MovementStatus_MovementStatus/1
  message_unpack/103(IFC_Line01_DxEnd) -> IFC_Line01_DxEnd_IFC_Line01_DxEnd/1
  vehicle_long_acc_in/1 -> vehicle_long_acc/1  "vehicle_long_acc"
  message_unpack/130(IFC_Line03_HeadingAngle) -> IFC_Line03_HeadingAngle_IFC_Line03_HeadingAngle/1
  CAFDva_y_F_CameraData425/1 -> message_unpack/28(CAFDva_y_F_CameraData425)
  CAFDva_y_F_CameraData450/1 -> message_unpack/29(CAFDva_y_F_CameraData450)
  message_unpack/120(IFC_Line02_Curv) -> IFC_Line02_Curv_IFC_Line02_Curv/1
  message_unpack/6(Radar_P_latd) -> LatDistance_LatDistance/1
  message_unpack/97(IFC_obj_DirIndicator) -> IFC_obj_DirIndicator_IFC_obj_DirIndicator/1
  message_unpack/96(IFC_obj_TTIPC) -> IFC_obj_TTIPC_IFC_obj_TTIPC/1
  message_unpack/163(IFC_Roadedge02_DxStart) -> IFC_Roadedge02_DxStart_IFC_Roadedge02_DxStart/1
  message_unpack/105(IFC_Line01_Dy) -> IFC_Line01_Dy_IFC_Line01_Dy/1
  message_unpack/51(FS_Blur_Image_0) -> FS_Blur_Image_0/1
  message_unpack/5(Radar_P_long_std) -> LongDistanceSTD_LongDistanceSTD/1
  message_unpack/58(IFC_obj_abs_Ay) -> IFC_obj_abs_Ay_IFC_obj_abs_Ay/1
  message_unpack/131(IFC_Line03_Dy) -> IFC_Line03_Dy_IFC_Line03_Dy/1
  message_unpack/3(Radar_num) -> NumberOfObj_NumberOfObj/1
